simulink model "sampleModel2022"  (R2023a)
settings: Solver=VariableStepAuto  StartTime=0.0  StopTime=10.0  RelTol=1e-3
libraries: hdlsllib x3
settings Model: Creator=user1  LastModifiedBy=user1

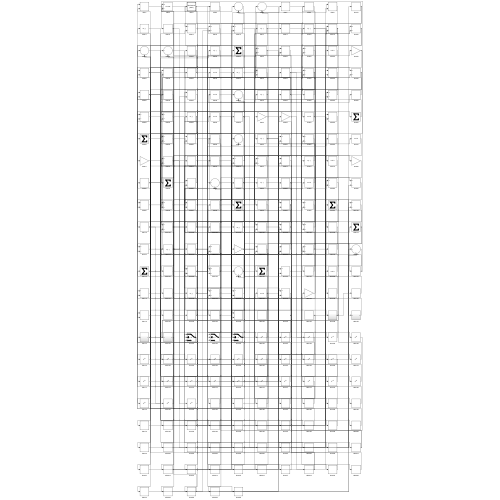
[thumbnail: Simulink's stored preview of the top-level diagram]
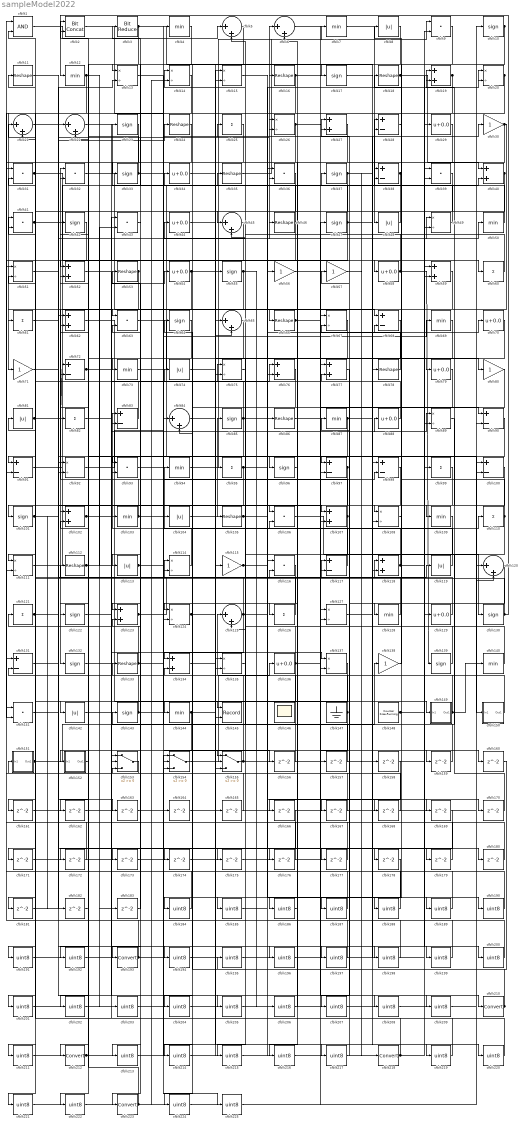
== system sampleModel2022 ==
  cfblk1 : Logic  AllPortsSameDT=off  OutDataTypeStr=boolean
  cfblk{10,17,23,33,37,42,47,55,64,85,96,101,122,130,132,139,143} (17 alike) : Signum
  cfblk{28,38,68,72,83,90..91,97..98,100,117,131} (12 alike) : Sum  Inputs=+-
  cfblk{19,27,40,52,59,62,76..77,102,107,118,123,134} (13 alike) : Sum
  cfblk{4,7,12,50,69,73,87,94,103,109,128,140,144} (13 alike) : MinMax
  cfblk{8,48,74,81,104,113,119,142} (8 alike) : Abs  SaturateOnIntegerOverflow=off
  cfblk{11,16,18,24,35,46,53,66,78,86,105,112,133} (13 alike) : Reshape
  cfblk{9,31..32,36,39,41,43,63,93,106,116,141} (12 alike) : DotProduct  OutDataTypeStr=Inherit: Inherit via internal rule
  cfblk{13..15,20,26,49,51,67,75,89,92,108,111,114,124,127,135,137} (18 alike) : Product  Inputs=*/  RndMeth=Zero  SaturateOnIntegerOverflow=on
  cfblk{25,60..61,82,95,99,110,121,126} (9 alike) : Sum  Inputs=+
  cfblk{30,56..57,71,80,115,138} (7 alike) : Gain
  cfblk{5..6,21..22,45,65,84,120,125} (9 alike) : Sum  Inputs=|++
  cfblk{29,34,44,54,58,70,79,88,129,136} (10 alike) : Bias  Bias=0.0  SaturateOnIntegerOverflow=off
  cfblk145 : Record  FileSettingsInternal="{\"entries\":[{\"content\":{\"excelSettings\":{\"content\":{},\"type\":\"Streamout.ExcelSettings\"}},\"type\":\"Streamout.FileSettingStorage\",\"uuid\":\"\"}],\"packageUris\":[\"http:\\/\\/schema.mathworks.com\\/mf0\\/streamout_blocks\\/R2020a\"],\"version\":\"1.0\"}"  Layout=[1 1]  SignalsInternal="{\"entries\":[{\"content\":{\"signals\":[{\"content\":{\"blockPath\":[],\"dimensions\":[1],\"domain\":\"\",\"lineColor\":\"#a2142f\",\"plots\":[1],\"port\":1,\"signalID\":6095,\"signalName\":\"XY Graph:1\"},\"type\":\"RecordBlkView.Signal\",\"uuid\":\"\"},{\"content\":{\"blockPath\":[],\"dimensions\":[1],\"domain\":\"\",\"lineColor\":\"#139fff\",\"plots\":[1],\"port\":2,\"signalID\":6098,\"signalName\":\"XY Graph:2\"},\"type\":\"RecordBlkView.Signal\",\"uuid\":\"\"}]},\"type\":\"RecordBlkView.InputSignals\",\"uuid\":\"\"}],\"packageUris\":[\"http:\\/\\/schema.mathworks.com\\/mf0\\/streamout_blocks\\/R2020a\"],\"version\":\"1.0\"}"  VisualizationBindings="{\"xyplotplugin\":{\"info\":[{\"series\":[{\"bindingParametersList\":[{\"parameter\":\"X-Axis\",\"signalID\":6095,\"signalName\":\"XY Graph:1\"},{\"parameter\":\"Y-Axis\",\"signalID\":6098,\"signalName\":\"XY Graph:2\"}],\"seriesID\":13059}],\"subplotID\":1}]}}"  CompatibilityTag=XY  st=-1
  cfblk146 : Scope
      settings: Floating=on
  cfblk147 : Ground
  cfblk148 : hdlsllib/Sources/Counter Free-Running  NumBits=16  tsamp=-1
  cfblk149 : Subsystem
      settings: LibrarySourceBlock=|
      | hdlsllib/Ports &
      | Subsystems/Subsystem
  cfblk150 : Subsystem
      settings: LibrarySourceBlock=|
      | hdlsllib/Ports &
      | Subsystems/Subsystem
  cfblk151 : Subsystem
      settings: LibrarySourceBlock=|
      | hdlsllib/Ports &
      | Subsystems/Subsystem
  cfblk152 : Subsystem
      settings: LibrarySourceBlock=|
      | hdlsllib/Ports &
      | Subsystems/Subsystem
  cfblk153 : Switch  SaturateOnIntegerOverflow=off  InputSameDT=off
  cfblk154 : Switch  SaturateOnIntegerOverflow=off  InputSameDT=off
  cfblk155 : Switch  SaturateOnIntegerOverflow=off  InputSameDT=off
  cfblk{156..183} (28 alike) : Delay  SampleTime=1
  cfblk{184..192,194..209,211,213..217,219..222,224..225} (37 alike) : DataTypeConversion  OutDataTypeStr=uint8  SaturateOnIntegerOverflow=off  RndMeth=Floor
  cfblk{193,210,212,218,223} (5 alike) : DataTypeConversion  SaturateOnIntegerOverflow=off  RndMeth=Floor
  cfblk2 : hdlsllib/Logic and Bit Operations/Bit Concat  numInputs=2
  cfblk3 : hdlsllib/Logic and Bit Operations/Bit Reduce  mode=AND
  wires:
  cfblk31/1 -> cfblk58/1, cfblk174/1
  cfblk136/1 -> cfblk44/1, cfblk145/2, cfblk168/1, cfblk216/1
  cfblk94/1 -> cfblk7/1
  cfblk50/1 -> cfblk23/1
  cfblk62/1 -> cfblk149/1(In1)
  cfblk118/1 -> cfblk83/1, cfblk20/2
  cfblk110/1 -> cfblk143/1, cfblk38/2, cfblk118/2
  cfblk30/1 -> cfblk66/1, cfblk171/1
  cfblk126/1 -> cfblk114/1
  cfblk7/1 -> cfblk48/1
  cfblk91/1 -> cfblk63/1
  cfblk70/1 -> cfblk125/1
  cfblk14/1 -> cfblk71/1
  cfblk119/1 -> cfblk94/1
  cfblk8/1 -> cfblk17/1
  cfblk27/1 -> cfblk106/1
  cfblk32/1 -> cfblk86/1
  cfblk114/1 -> cfblk83/2
  cfblk107/1 -> cfblk32/1, cfblk175/1
  cfblk45/1 -> cfblk134/1
  cfblk88/1 -> cfblk32/2
  cfblk123/1 -> cfblk117/1, cfblk98/2, cfblk25/1
  cfblk54/1 -> cfblk123/1, cfblk79/1
  cfblk39/1 -> cfblk193/1
  cfblk22/1 -> cfblk60/1
  cfblk130/1 -> cfblk12/1, cfblk21/2
  cfblk53/1 -> cfblk132/1, cfblk61/1
  cfblk48/1 -> cfblk45/1
  cfblk111/1 -> cfblk6/1
  cfblk4/1 -> cfblk102/1
  cfblk58/1 -> cfblk139/1, cfblk34/1
  cfblk33/1 -> cfblk2/1, cfblk27/1
  cfblk96/1 -> cfblk126/1
  cfblk35/1 -> cfblk9/1
  cfblk60/1 -> cfblk16/1
  cfblk154/1 -> cfblk136/1
  cfblk49/1 -> cfblk28/1
  cfblk40/1 -> cfblk137/2, cfblk221/1
  cfblk80/1 -> cfblk145/1
  cfblk129/1 -> cfblk1/2
  cfblk24/1 -> cfblk122/1
  cfblk73/1 -> cfblk35/1
  cfblk63/1 -> cfblk150/1(In1)
  cfblk138/1 -> cfblk18/1
  cfblk148/1 -> cfblk129/1, cfblk188/1
  cfblk106/1 -> cfblk130/1
  cfblk133/1 -> cfblk110/1, cfblk118/1, cfblk31/2
  cfblk135/1 -> cfblk75/1
  cfblk10/1 -> cfblk108/1, cfblk155/2
  cfblk104/1 -> cfblk85/1
  cfblk134/1 -> cfblk105/1
  cfblk155/1 -> cfblk53/1, cfblk49/2
  cfblk65/1 -> cfblk212/1
  cfblk81/1 -> cfblk72/1, cfblk93/2
  cfblk38/1 -> cfblk82/1, cfblk166/1
  cfblk83/1 -> cfblk21/1
  cfblk42/1 -> cfblk101/1
  cfblk75/1 -> cfblk45/2
  cfblk139/1 -> cfblk14/1
  cfblk56/1 -> cfblk210/1
  cfblk66/1 -> cfblk169/1, cfblk170/1
  cfblk19/1 -> cfblk128/1, cfblk124/2
  cfblk78/1 -> cfblk37/1
  cfblk3/1 -> cfblk98/1, cfblk13/1
  cfblk89/1 -> cfblk109/1
  cfblk2/1 -> cfblk84/1
  cfblk64/1 -> cfblk142/1
  cfblk132/1 -> cfblk89/1
  cfblk16/1 -> cfblk90/1, cfblk211/1
  cfblk142/1 -> cfblk88/1
  cfblk47/1 -> cfblk26/1, cfblk111/2, cfblk6/2, cfblk189/1
  cfblk150/1(Out1) -> cfblk62/2
  cfblk23/1 -> cfblk33/1
  cfblk41/1 -> cfblk38/1, cfblk13/2, cfblk107/1
  cfblk108/1 -> cfblk8/1
  cfblk144/1 -> cfblk50/1, cfblk202/1
  cfblk100/1 -> cfblk223/1
  cfblk115/1 -> cfblk19/1, cfblk70/1
  cfblk18/1 -> cfblk40/1, cfblk200/1
  cfblk52/1 -> cfblk137/1
  cfblk125/1 -> cfblk52/2, cfblk154/3, cfblk167/1
  cfblk69/1 -> cfblk73/1
  cfblk21/1 -> cfblk26/2
  cfblk46/1 -> cfblk3/1, cfblk93/1
  cfblk147/1 -> cfblk154/2, cfblk121/1
  cfblk122/1 -> cfblk119/1
  cfblk72/1 -> cfblk96/1, cfblk203/1
  cfblk103/1 -> cfblk22/2, cfblk49/1, cfblk155/1
  cfblk5/1 -> cfblk144/1
  cfblk20/1 -> cfblk108/2, cfblk213/1
  cfblk84/1 -> cfblk115/1
  cfblk68/1 -> cfblk125/2
  cfblk13/1 -> cfblk68/1
  cfblk87/1 -> cfblk30/1, cfblk152/1(In1)
  cfblk34/1 -> cfblk80/1
  cfblk140/1 -> cfblk68/2
  cfblk151/1(Out1) -> cfblk4/1, cfblk138/1
  cfblk90/1 -> cfblk153/2
  cfblk9/1 -> cfblk113/1
  cfblk92/1 -> cfblk40/2
  cfblk101/1 -> cfblk41/1, cfblk46/1, cfblk182/1
  cfblk105/1 -> cfblk28/2, cfblk185/1
  cfblk57/1 -> cfblk218/1
  cfblk29/1 -> cfblk141/2
  cfblk121/1 -> cfblk114/2, cfblk24/1
  cfblk143/1 -> cfblk131/2, cfblk69/1
  cfblk25/1 -> cfblk91/1
  cfblk128/1 -> cfblk103/1
  cfblk76/1 -> cfblk124/1
  cfblk153/1 -> cfblk151/1(In1)
  cfblk12/1 -> cfblk91/2, cfblk183/1
  cfblk95/1 -> cfblk135/2, cfblk20/1
  cfblk112/1 -> cfblk76/1, cfblk43/2, cfblk180/1
  cfblk26/1 -> cfblk52/1, cfblk160/1
  cfblk124/1 -> cfblk104/1, cfblk209/1
  cfblk55/1 -> cfblk111/1, cfblk206/1
  cfblk149/1(Out1) -> cfblk95/1, cfblk140/1
  cfblk97/1 -> cfblk155/3, cfblk191/1
  cfblk113/1 -> cfblk156/1, cfblk217/1
  cfblk86/1 -> cfblk47/1
  cfblk102/1 -> cfblk54/1, cfblk208/1
  cfblk1/1 -> cfblk5/1
  cfblk117/1 -> cfblk106/2
  cfblk37/1 -> cfblk92/2, cfblk158/1, cfblk159/1
  cfblk82/1 -> cfblk74/1
  cfblk79/1 -> cfblk89/2
  cfblk85/1 -> cfblk72/2, cfblk97/1, cfblk214/1
  cfblk156/1 -> cfblk84/2
  cfblk157/1 -> cfblk63/2
  cfblk159/1 -> cfblk5/2
  cfblk137/1 -> cfblk161/1
  cfblk161/1 -> cfblk90/2
  cfblk99/1 -> cfblk162/1
  cfblk162/1 -> cfblk153/1
  cfblk71/1 -> cfblk163/1
  cfblk163/1 -> cfblk75/2
  cfblk164/1 -> cfblk134/2
  cfblk74/1 -> cfblk165/1
  cfblk165/1 -> cfblk135/1
  cfblk167/1 -> cfblk92/1
  cfblk168/1 -> cfblk1/1
  cfblk170/1 -> cfblk19/2
  cfblk171/1 -> cfblk97/2
  cfblk152/1(Out1) -> cfblk172/1
  cfblk172/1 -> cfblk131/1
  cfblk43/1 -> cfblk173/1
  cfblk173/1 -> cfblk154/1
  cfblk174/1 -> cfblk107/2
  cfblk175/1 -> cfblk76/2
  cfblk109/1 -> cfblk176/1
  cfblk176/1 -> cfblk102/2
  cfblk61/1 -> cfblk177/1
  cfblk177/1 -> cfblk62/1
  cfblk28/1 -> cfblk178/1
  cfblk17/1 -> cfblk179/1
  cfblk179/1 -> cfblk117/2
  cfblk180/1 -> cfblk153/3
  cfblk98/1 -> cfblk181/1
  cfblk181/1 -> cfblk22/1
  cfblk182/1 -> cfblk2/2
  cfblk183/1 -> cfblk123/2
  cfblk36/1 -> cfblk184/1
  cfblk184/1 -> cfblk133/1
  cfblk185/1 -> cfblk36/1
  cfblk158/1 -> cfblk186/1
  cfblk186/1 -> cfblk36/2
  cfblk77/1 -> cfblk187/1
  cfblk187/1 -> cfblk31/1
  cfblk188/1 -> cfblk77/1
  cfblk189/1 -> cfblk77/2
  cfblk15/1 -> cfblk190/1
  cfblk190/1 -> cfblk41/2
  cfblk191/1 -> cfblk15/1
  cfblk166/1 -> cfblk192/1
  cfblk192/1 -> cfblk15/2
  cfblk193/1 -> cfblk42/1, cfblk78/1, cfblk197/1
  cfblk131/1 -> cfblk194/1
  cfblk194/1 -> cfblk39/1
  cfblk160/1 -> cfblk195/1
  cfblk195/1 -> cfblk39/2
  cfblk51/1 -> cfblk196/1
  cfblk196/1 -> cfblk9/2
  cfblk197/1 -> cfblk51/1
  cfblk6/1 -> cfblk198/1
  cfblk198/1 -> cfblk51/2
  cfblk11/1 -> cfblk199/1
  cfblk199/1 -> cfblk141/1
  cfblk200/1 -> cfblk11/1
  cfblk59/1 -> cfblk201/1
  cfblk201/1 -> cfblk55/1
  cfblk202/1 -> cfblk59/1
  cfblk203/1 -> cfblk59/2
  cfblk116/1 -> cfblk204/1
  cfblk204/1 -> cfblk99/1
  cfblk141/1 -> cfblk205/1
  cfblk205/1 -> cfblk116/1
  cfblk206/1 -> cfblk116/2
  cfblk120/1 -> cfblk207/1
  cfblk207/1 -> cfblk10/1
  cfblk208/1 -> cfblk120/1
  cfblk209/1 -> cfblk120/2
  cfblk210/1 -> cfblk27/2, cfblk64/1
  cfblk211/1 -> cfblk56/1
  cfblk212/1 -> cfblk164/1, cfblk29/1
  cfblk213/1 -> cfblk65/1
  cfblk214/1 -> cfblk65/2
  cfblk67/1 -> cfblk215/1
  cfblk215/1 -> cfblk157/1
  cfblk216/1 -> cfblk67/1
  cfblk217/1 -> cfblk67/2
  cfblk218/1 -> cfblk43/1, cfblk87/1
  cfblk44/1 -> cfblk219/1
  cfblk219/1 -> cfblk57/1
  cfblk127/1 -> cfblk220/1
  cfblk220/1 -> cfblk81/1
  cfblk221/1 -> cfblk127/1
  cfblk169/1 -> cfblk222/1
  cfblk222/1 -> cfblk127/2
  cfblk223/1 -> cfblk112/1, cfblk14/2
  cfblk178/1 -> cfblk224/1
  cfblk224/1 -> cfblk100/1
  cfblk93/1 -> cfblk225/1
  cfblk225/1 -> cfblk100/2

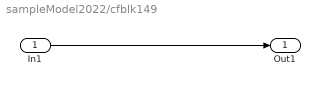
== system sampleModel2022/cfblk149 ==
  In1 : Inport
  Out1 : Outport
  wires:
  In1/1 -> Out1/1

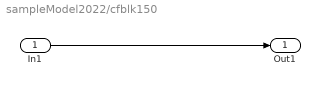
== system sampleModel2022/cfblk150 ==
  In1 : Inport
  Out1 : Outport
  wires:
  In1/1 -> Out1/1

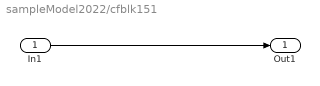
== system sampleModel2022/cfblk151 ==
  In1 : Inport
  Out1 : Outport
  wires:
  In1/1 -> Out1/1

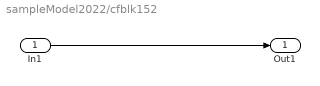
== system sampleModel2022/cfblk152 ==
  In1 : Inport
  Out1 : Outport
  wires:
  In1/1 -> Out1/1
